simulink model "mobilebot_Model"  (R2018a)
settings: Solver=VariableStepAuto  StartTime=0.0  StopTime=10.0  RelTol=1e-3
libraries: simulink x1
settings Model: Creator=ewolbrec  LastModifiedBy=nalha
settings CodeAppCC: StateflowObjectComments=on

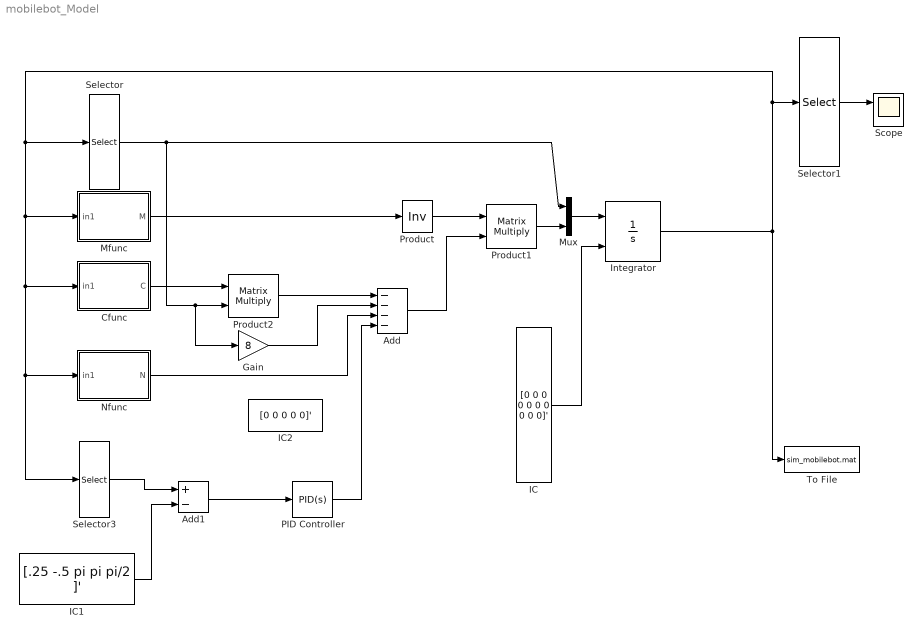
== system mobilebot_Model ==
  Add : Sum  Inputs=----
  Add1 : Sum  Inputs=+-
  Cfunc : MATLAB Function  TreatAsAtomicUnit=on
  Gain : Gain  Gain=8
  IC : Constant  Value=[0 0 0 0 0 0 0 0 0 0]'  VectorParams1D=off
  IC1 : Constant  Value=[.25 -.5 pi pi pi/2 ]'  VectorParams1D=off
  IC2 : Constant  Value=[0 0 0 0 0]'  VectorParams1D=off
  Integrator : Integrator  InitialConditionSource=external
  Mfunc : MATLAB Function  TreatAsAtomicUnit=on
  Mux : Mux  Inputs=2
  Nfunc : MATLAB Function  TreatAsAtomicUnit=on
  PID Controller : simulink/Continuous/PID Controller  Controller=PID  TimeDomain=Continuous-time  SampleTime=-1  IntegratorMethod=Forward Euler  FilterMethod=Forward Euler  Form=Parallel  UseFilter=on  ControllerParametersSource=internal  P=200  I=25  D=70  N=150  InitialConditionSource=internal  InitialConditionForIntegrator=0  InitialConditionForFilter=0  ExternalReset=none  LimitOutput=off  UpperSaturationLimit=inf  LowerSaturationLimit=-inf  LinearizeAsGain=on  AntiWindupMode=none  Kb=1  TrackingMode=off  Kt=1  PParamMin=[]  PParamMax=[]  IParamMin=[]  IParamMax=[]  DParamMin=[]  DParamMax=[]  NParamMin=[]  NParamMax=[]  KbParamMin=[]  KbParamMax=[]  KtParamMin=[]  KtParamMax=[]  POutMin=[]  POutMax=[]  IOutMin=[]  IOutMax=[]  DOutMin=[]  DOutMax=[]  NOutMin=[]  NOutMax=[]  KbOutMin=[]  KbOutMax=[]  KtOutMin=[]  KtOutMax=[]  IntegratorOutMin=[]  IntegratorOutMax=[]  FilterOutMin=[]  FilterOutMax=[]  SumOutMin=[]  SumOutMax=[]  SumI1OutMin=[]  SumI1OutMax=[]  SumI2OutMin=[]  SumI2OutMax=[]  SumI3OutMin=[]  SumI3OutMax=[]  SumDOutMin=[]  SumDOutMax=[]  SaturationOutMin=[]  SaturationOutMax=[]  IntegratorContinuousStateAttributes=''  IntegratorStateMustResolveToSignalObject=off  IntegratorRTWStateStorageClass=Auto  FilterContinuousStateAttributes=''  FilterStateMustResolveToSignalObject=off  FilterRTWStateStorageClass=Auto  DifferentiatorICPrevScaledInput=0  DifferentiatorOutMin=[]  DifferentiatorOutMax=[]  FilterDiffOutCoefMin=[]  FilterDiffOutCoefMax=[]  SumDenOutMin=[]  SumDenOutMax=[]  SumNumOutMin=[]  SumNumOutMax=[]  ReciprocalOutMin=[]  ReciprocalOutMax=[]  DivideOutMin=[]  DivideOutMax=[]  TunerSelectOption=Transfer Function Based (PID Tuner App)
  Product : Product  Inputs=/  Multiplication=Matrix(*)
  Product1 : Product  Inputs=**  Multiplication=Matrix(*)
  Product2 : Product  Inputs=**  Multiplication=Matrix(*)
  Scope : Scope  NumInputPorts=2
  Selector : Selector  InputPortWidth=10  IndexOptions=Index vector (dialog)  Indices=[6 7 8 9 10]  OutputSizes=1
  Selector1 : Selector  InputPortWidth=10  IndexOptions=Index vector (dialog)  Indices=[1 2 3 4 5]  OutputSizes=1
  Selector3 : Selector  InputPortWidth=10  IndexOptions=Index vector (dialog)  Indices=[1 2 3 4 5]  OutputSizes=1
  To File : ToFile  Filename=sim_mobilebot.mat  SampleTime=1/30
  wires:
  Mfunc/1(M) -> Product/1
  Mux/1 -> Integrator/1
  Product1/1 -> Mux/2
  Selector/1 -> Gain/1, Product2/2, Mux/1
  Cfunc/1(C) -> Product2/1
  Product/1 -> Product1/1
  Gain/1 -> Add/2
  Product2/1 -> Add/1
  Nfunc/1(N) -> Add/3
  Add/1 -> Product1/2
  IC/1 -> Integrator/2
  Selector1/1 -> Scope/1
  Selector3/1 -> Add1/1
  IC1/1 -> Add1/2
  Add1/1 -> PID Controller/1
  Integrator/1 -> To File/1, Mfunc/1(in1), Cfunc/1(in1), Selector3/1, Nfunc/1(in1), Selector/1, Selector1/1
  PID Controller/1 -> Add/4

== matlab function mobilebot_Model/Cfunc ==
  data: in1 input; C output
function C = Cfunc(in1)
%#codegen

%    This function was generated by the Symbolic Math Toolbox version 8.1.
%    08-May-2018 14:55:47

th3 = in1(3,:);
th4 = in1(4,:);
th5 = in1(5,:);
th3d = in1(8,:);
th4d = in1(9,:);
th5d = in1(10,:);
t2 = cos(th3);
t3 = cos(th4);
t4 = sin(th3);
t5 = cos(th5);
t6 = sin(th4);
t7 = sin(th5);
t8 = t2.*t3.*t7.*th3d.*(2.7e1./8.0);
t9 = t2.*t5.*t6.*th3d.*(2.7e1./8.0);
t10 = t3.*t4.*t5.*th4d.*(2.7e1./8.0);
t11 = t3.*t4.*t5.*th5d.*(2.7e1./8.0);
t12 = t3.*t4.*t7.*th3d.*(2.7e1./8.0);
t13 = t4.*t5.*t6.*th3d.*(2.7e1./8.0);
t14 = t2.*t6.*t7.*th4d.*(2.7e1./8.0);
t15 = t2.*t6.*t7.*th5d.*(2.7e1./8.0);
t16 = th4.*2.0;
t17 = th5.*2.0;
t18 = t16+t17;
t19 = sin(t18);
t20 = t16+th5;
t21 = sin(t20);
t22 = sin(t16);
t23 = th4+th5;
t24 = cos(t23);
t25 = t19.*3.3e1;
C = reshape([0.0,0.0,0.0,0.0,0.0,0.0,0.0,0.0,0.0,0.0,t2.*th3d.*(-2.7e1./1.0e1)+t3.*t4.*th3d.*(8.1e1./8.0)+t2.*t6.*th4d.*(8.1e1./8.0)+t3.*t4.*t5.*th3d.*(2.7e1./8.0)+t2.*t3.*t7.*th4d.*(2.7e1./8.0)+t2.*t3.*t7.*th5d.*(2.7e1./8.0)+t2.*t5.*t6.*th4d.*(2.7e1./8.0)+t2.*t5.*t6.*th5d.*(2.7e1./8.0)-t4.*t6.*t7.*th3d.*(2.7e1./8.0),t4.*th3d.*(-2.7e1./1.0e1)-t2.*t3.*th3d.*(8.1e1./8.0)+t4.*t6.*th4d.*(8.1e1./8.0)-t2.*t3.*t5.*th3d.*(2.7e1./8.0)+t2.*t6.*t7.*th3d.*(2.7e1./8.0)+t3.*t4.*t7.*th4d.*(2.7e1./8.0)+t3.*t4.*t7.*th5d.*(2.7e1./8.0)+t4.*t5.*t6.*th4d.*(2.7e1./8.0)+t4.*t5.*t6.*th5d.*(2.7e1./8.0),t7.*th5d.*(-2.7e1./3.2e1)-t19.*th4d.*5.56875e-1-t19.*th5d.*5.56875e-1-t21.*th4d.*(2.7e1./1.6e1)-t21.*th5d.*(2.7e1./3.2e1)-t22.*th4d.*2.244375,th3d.*(t21.*1.0e2+t22.*1.33e2+t25).*1.6875e-2,th3d.*(t7.*5.0e1+t21.*5.0e1+t25).*1.6875e-2,t8+t9+t10+t11+t2.*t6.*th3d.*(8.1e1./8.0)+t3.*t4.*th4d.*(8.1e1./8.0)-t4.*t6.*t7.*th4d.*(2.7e1./8.0)-t4.*t6.*t7.*th5d.*(2.7e1./8.0),t12+t13+t14+t15-t2.*t3.*th4d.*(8.1e1./8.0)+t4.*t6.*th3d.*(8.1e1./8.0)-t2.*t3.*t5.*th4d.*(2.7e1./8.0)-t2.*t3.*t5.*th5d.*(2.7e1./8.0),t3.*th4d.*(-8.1e1./8.0e1)-t19.*th3d.*5.56875e-1-t21.*th3d.*(2.7e1./1.6e1)-t22.*th3d.*2.244375-t24.*th4d.*(2.7e1./8.0e1)-t24.*th5d.*(2.7e1./8.0e1),t7.*th5d.*(-2.7e1./1.6e1),t7.*th4d.*(2.7e1./1.6e1),t8+t9+t10+t11-t4.*t6.*t7.*th4d.*(2.7e1./8.0)-t4.*t6.*t7.*th5d.*(2.7e1./8.0),t12+t13+t14+t15-t2.*t3.*t5.*th4d.*(2.7e1./8.0)-t2.*t3.*t5.*th5d.*(2.7e1./8.0),t7.*th3d.*(-2.7e1./3.2e1)-t19.*th3d.*5.56875e-1-t21.*th3d.*(2.7e1./3.2e1)-t24.*th4d.*(2.7e1./8.0e1)-t24.*th5d.*(2.7e1./8.0e1),t7.*(th4d+th5d).*(-2.7e1./1.6e1),0.0],[5,5]);

== matlab function mobilebot_Model/Mfunc ==
  data: in1 input; M output
function M = Mfunc(in1)
%#codegen

%    This function was generated by the Symbolic Math Toolbox version 8.1.
%    08-May-2018 14:55:47

th3 = in1(3,:);
th4 = in1(4,:);
th5 = in1(5,:);
t2 = cos(th3);
t3 = cos(th4);
t4 = sin(th3);
t5 = sin(th4);
t6 = th4+th5;
t7 = sin(t6);
t8 = sin(th5);
t9 = cos(th5);
t10 = t5.*3.0;
t11 = t7+t10;
t12 = t2.*t5.*t8.*(2.7e1./8.0);
t13 = t4.*(-2.7e1./1.0e1)+t12-t2.*t3.*(8.1e1./8.0)-t2.*t3.*t9.*(2.7e1./8.0);
t14 = t2.*(2.7e1./1.0e1);
t15 = t4.*t5.*t8.*(2.7e1./8.0);
t16 = t14+t15-t3.*t4.*(8.1e1./8.0)-t3.*t4.*t9.*(2.7e1./8.0);
t17 = th4.*2.0;
t18 = t4.*t11.*(2.7e1./8.0);
t22 = t7.*(2.7e1./8.0e1);
t19 = t5.*(-8.1e1./8.0e1)-t22;
t20 = t9.*(2.7e1./1.6e1);
t21 = t4.*t7.*(2.7e1./8.0);
t23 = t20+9.07e2./8.0e2;
M = reshape([7.83e2./5.0,0.0,t13,t18,t21,0.0,7.83e2./5.0,t16,t2.*t11.*(-2.7e1./8.0),t2.*t7.*(-2.7e1./8.0),t13,t16,t20+cos(t17+th5.*2.0).*5.56875e-1+cos(t17+th5).*(2.7e1./1.6e1)+cos(t17).*2.244375+6.57125,t19,-t22,t18,t2.*t11.*(-2.7e1./8.0),t19,t9.*(2.7e1./8.0)+5.6425,t23,t21,t2.*t7.*(-2.7e1./8.0),t7.*(-2.7e1./8.0e1),t23,9.07e2./8.0e2],[5,5]);

== matlab function mobilebot_Model/Nfunc ==
  data: in1 input; N output
function N = Nfunc(in1)
%#codegen

%    This function was generated by the Symbolic Math Toolbox version 8.1.
%    08-May-2018 14:55:47

th4 = in1(4,:);
th5 = in1(5,:);
t2 = th4+th5;
t3 = cos(t2);
N = [0.0;0.0;0.0;t3.*(-1.35e2./4.0)-cos(th4).*(4.05e2./4.0);t3.*(-1.35e2./4.0)];
